simulink subsystem "microController"  (R2022b)
settings: Solver=VariableStepAuto  StartTime=0.0  StopTime=10.0  RelTol=1e-3
values from neighbouring files (symbols this model uses):
  Ts = 1/f    (= 5e-06)    [BLDCmotor.m]
  Ts_ctrl = 1/f_ctrl    (= 6.25e-05)    [BLDCmotor.m]
  vec_hallToPos = [0 2 0 1 4 3 5 0]    [BLDCmotor.m]
  Vs = motor.Vs    [BLDCmotor.m]    (also in geraModeloHover.m = 36)
libraries: slpidlib x3, spsPWMGeneratorDCDCLib x3
settings Model: Creator=hemil  LastModifiedBy=hemil

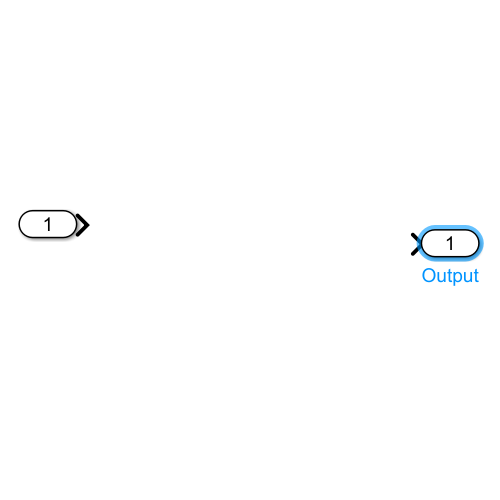
[thumbnail: Simulink's stored preview of the top-level diagram]
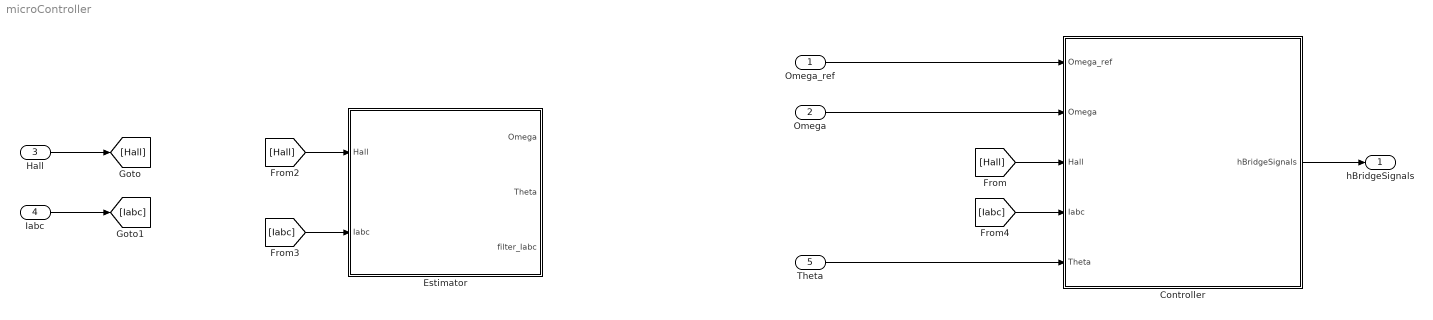
== system microController ==
  Omega_ref : Inport
  Omega : Inport  Port=2
  Hall : Inport  Port=3
  Iabc : Inport  Port=4
  Theta : Inport  Port=5
  Controller : Subsystem  Variant=on
  Estimator : Subsystem
  hBridgeSignals : Outport
  wires:
  Omega_ref/1 -> Controller/1(Omega_ref)
  Omega/1 -> Controller/2(Omega)
  Hall/1 -> [Hall]
  [Iabc] -> Controller/4(Iabc)
  Controller/1(hBridgeSignals) -> hBridgeSignals/1
  Theta/1 -> Controller/5(Theta)
  [Hall] -> Controller/3(Hall)
  [Hall] -> Estimator/1(Hall)
  Iabc/1 -> [Iabc]
  [Iabc] -> Estimator/2(Iabc)

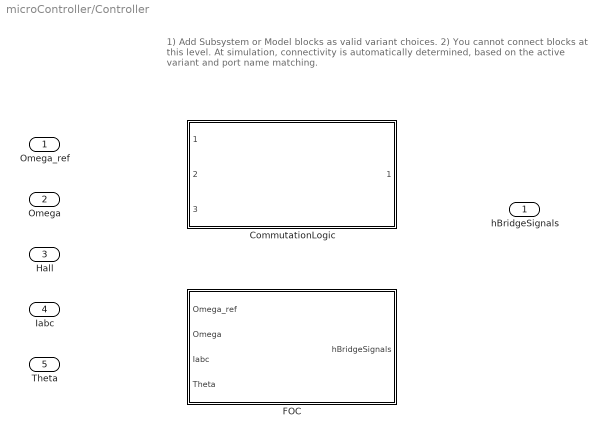
== system microController/Controller ==
  note: 1) Add Subsystem or Model blocks as valid variant choices.
      | 2) You cannot connect blocks at this level. At simulation, connectivity is automatically
      | determined, based on the active variant and port name matching.
  Omega_ref : Inport
  Omega : Inport  Port=2
  Hall : Inport  Port=3
  Iabc : Inport  Port=4
  Theta : Inport  Port=5
  CommutationLogic : Subsystem  VariantControl=(default)  ReferencedSubsystem=commutationLogic
  FOC : Subsystem  VariantControl=ControlMode == 1
  hBridgeSignals : Outport

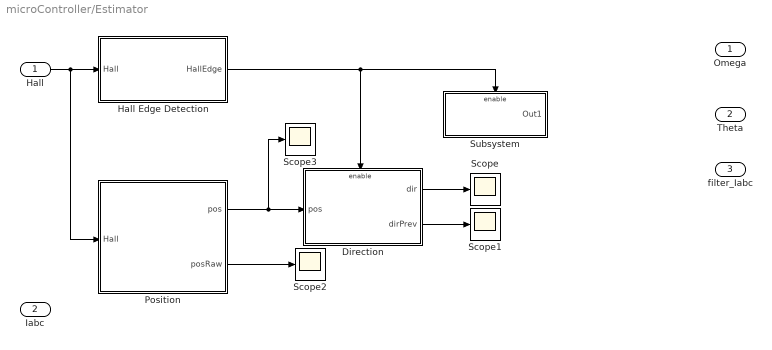
== system microController/Estimator ==
  Hall : Inport
  Iabc : Inport  Port=2
  Direction : Subsystem
  Hall Edge Detection : Subsystem
  Position : Subsystem
  Scope{,1..3} (4 alike) : Scope
  Subsystem : Subsystem
  Omega : Outport
  Theta : Outport  Port=2
  filter_Iabc : Outport  Port=3
  wires:
  Position/2(posRaw) -> Scope2/1
  Direction/2(dirPrev) -> Scope1/1
  Direction/1(dir) -> Scope/1
  Position/1(pos) -> Direction/1(pos), Scope3/1
  Hall/1 -> Hall Edge Detection/1(Hall), Position/1(Hall)
  Hall Edge Detection/1(HallEdge) -> Direction/Enable, Subsystem/Enable

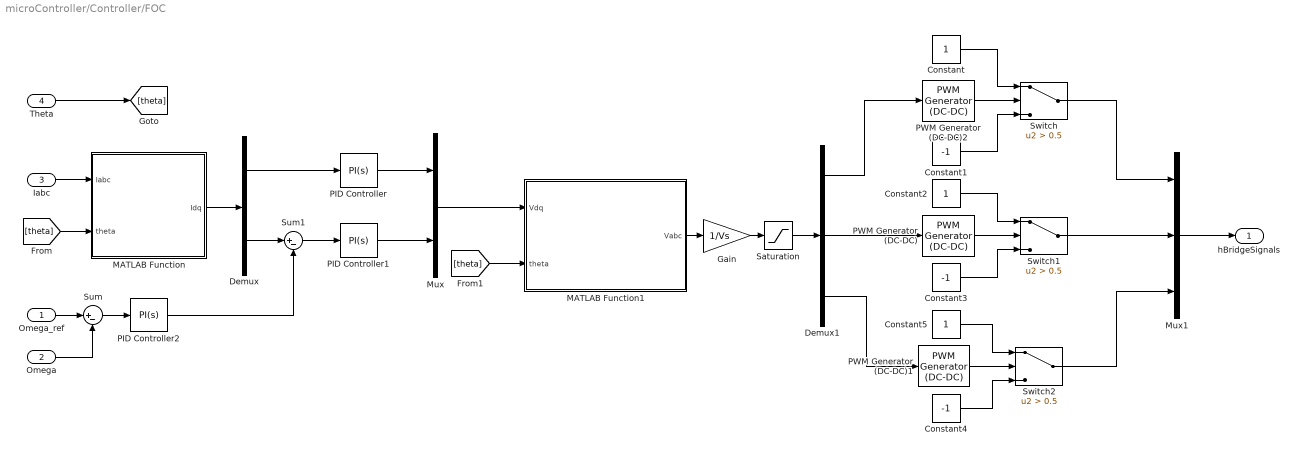
== system microController/Controller/FOC ==
  Omega_ref : Inport
  Omega : Inport  Port=2
  Iabc : Inport  Port=3
  Theta : Inport  Port=4
  Constant : Constant
  Constant1 : Constant  Value=-1
  Constant2 : Constant
  Constant3 : Constant  Value=-1
  Constant4 : Constant  Value=-1
  Constant5 : Constant
  Demux : Demux  Outputs=2
  Demux1 : Demux  Outputs=3
  Gain : Gain  Gain=1/Vs
  MATLAB Function : MATLAB Function  TreatAsAtomicUnit=on
  MATLAB Function1 : MATLAB Function  TreatAsAtomicUnit=on
  Mux : Mux  Inputs=2
  Mux1 : Mux  Inputs=3
  PID Controller : slpidlib/PID Controller  Controller=PI  Form=Parallel  TimeDomain=Continuous-time  UseExternalTs=off  SampleTime=-1  IntegratorMethod=Forward Euler  FilterMethod=Forward Euler  ControllerParametersSource=internal  P=1  I=0.1  UseKiTs=off  D=0  N=100  UseFilter=on  TunerSelectOption=Transfer Function Based (PID Tuner App)  InitialConditionSource=internal  InitialConditionForIntegrator=0  InitialConditionForFilter=0  DifferentiatorICPrevScaledInput=0  ExternalReset=none  TrackingMode=off  Kt=1  LimitOutput=off  SatLimitsSource=internal  UpperSaturationLimit=inf  LowerSaturationLimit=-inf  LinearizeAsGain=on  AntiWindupMode=none  Kb=1  LimitIntegrator=off  UpperIntegratorSaturationLimit=inf  LowerIntegratorSaturationLimit=-inf  POutMin=[]  POutMax=[]  IOutMin=[]  IOutMax=[]  DOutMin=[]  DOutMax=[]  NOutMin=[]  NOutMax=[]  SumOutMin=[]  SumOutMax=[]  SaturationOutMin=[]  SaturationOutMax=[]  PParamMin=[]  PParamMax=[]  IParamMin=[]  IParamMax=[]  DParamMin=[]  DParamMax=[]  NParamMin=[]  NParamMax=[]  KbParamMin=[]  KbParamMax=[]  KtParamMin=[]  KtParamMax=[]  KbOutMin=[]  KbOutMax=[]  KtOutMin=[]  KtOutMax=[]  IntegratorOutMin=[]  IntegratorOutMax=[]  FilterOutMin=[]  FilterOutMax=[]  SumI1OutMin=[]  SumI1OutMax=[]  SumI2OutMin=[]  SumI2OutMax=[]  SumI3OutMin=[]  SumI3OutMax=[]  SumI4OutMin=[]  SumI4OutMax=[]  SumDOutMin=[]  SumDOutMax=[]  DifferentiatorOutMin=[]  DifferentiatorOutMax=[]  FilterDiffOutCoefMin=[]  FilterDiffOutCoefMax=[]  ReciprocalOutMin=[]  ReciprocalOutMax=[]  SumDenOutMin=[]  SumDenOutMax=[]  SumNumOutMin=[]  SumNumOutMax=[]  DivideOutMin=[]  DivideOutMax=[]  UdiffTsProdOutMin=[]  UdiffTsProdOutMax=[]  NTsProdOutMin=[]  NTsProdOutMax=[]  UintegralTsProdOutMin=[]  UintegralTsProdOutMax=[]  UngainTsProdOutMin=[]  UngainTsProdOutMax=[]  ClampingZeroOutDataTypeStr=Inherit: Inherit via back propagation  ClampingZeroOutMin=[]  ClampingZeroOutMax=[]  FilterDenConstantOutDataTypeStr=Inherit: Inherit via back propagation  FilterDenConstantOutMin=[]  FilterDenConstantOutMax=[]  PCopyOutDataTypeStr=Inherit: Inherit via back propagation  PCopyOutMin=[]  PCopyOutMax=[]  NCopyOutDataTypeStr=Inherit: Inherit via back propagation  NCopyOutMin=[]  NCopyOutMax=[]  IntegratorContinuousStateAttributes=''  IntegratorStateMustResolveToSignalObject=off  IntegratorRTWStateStorageClass=Auto  FilterContinuousStateAttributes=''  FilterStateMustResolveToSignalObject=off  FilterRTWStateStorageClass=Auto  ParallelPVariant=InternalParameters  IdealPVariant=Disabled  IVariant=InternalParameters  DVariant=Disabled  IntegratorVariant=Continuous  SatVariant=Disabled  AWVariant=Passthrough  PCopyVariant=Disabled  TRVariant=Disabled  FdbkBlocksVariant=Forward  IdealPFdbkVariant=Disabled  SatFdbkVariant=Disabled  DerivativeFilterVariant=Disabled  NVariant=Disabled  NCopyVariant=Disabled_SignalSpec  FilterICVariant=Disabled  IntegratorICVariant=InternalICs  ExternalResetVariant=Disabled  TRSumVariant=Passthrough  SumFdbkVariant=Disabled  SumVariant=Sum_PI  TsampFilterVariant=InternalTs  TsampNgainVariant=Passthrough  TsampIntegralVariant=Passthrough  ExternalSaturationOutDataTypeStr=Inherit: Same as second input
  PID Controller1 : slpidlib/PID Controller  Controller=PI  Form=Parallel  TimeDomain=Continuous-time  UseExternalTs=off  SampleTime=-1  IntegratorMethod=Forward Euler  FilterMethod=Forward Euler  ControllerParametersSource=internal  P=1  I=0.1  UseKiTs=off  D=0  N=100  UseFilter=on  TunerSelectOption=Transfer Function Based (PID Tuner App)  InitialConditionSource=internal  InitialConditionForIntegrator=0  InitialConditionForFilter=0  DifferentiatorICPrevScaledInput=0  ExternalReset=none  TrackingMode=off  Kt=1  LimitOutput=off  SatLimitsSource=internal  UpperSaturationLimit=inf  LowerSaturationLimit=-inf  LinearizeAsGain=on  AntiWindupMode=none  Kb=1  LimitIntegrator=off  UpperIntegratorSaturationLimit=inf  LowerIntegratorSaturationLimit=-inf  POutMin=[]  POutMax=[]  IOutMin=[]  IOutMax=[]  DOutMin=[]  DOutMax=[]  NOutMin=[]  NOutMax=[]  SumOutMin=[]  SumOutMax=[]  SaturationOutMin=[]  SaturationOutMax=[]  PParamMin=[]  PParamMax=[]  IParamMin=[]  IParamMax=[]  DParamMin=[]  DParamMax=[]  NParamMin=[]  NParamMax=[]  KbParamMin=[]  KbParamMax=[]  KtParamMin=[]  KtParamMax=[]  KbOutMin=[]  KbOutMax=[]  KtOutMin=[]  KtOutMax=[]  IntegratorOutMin=[]  IntegratorOutMax=[]  FilterOutMin=[]  FilterOutMax=[]  SumI1OutMin=[]  SumI1OutMax=[]  SumI2OutMin=[]  SumI2OutMax=[]  SumI3OutMin=[]  SumI3OutMax=[]  SumI4OutMin=[]  SumI4OutMax=[]  SumDOutMin=[]  SumDOutMax=[]  DifferentiatorOutMin=[]  DifferentiatorOutMax=[]  FilterDiffOutCoefMin=[]  FilterDiffOutCoefMax=[]  ReciprocalOutMin=[]  ReciprocalOutMax=[]  SumDenOutMin=[]  SumDenOutMax=[]  SumNumOutMin=[]  SumNumOutMax=[]  DivideOutMin=[]  DivideOutMax=[]  UdiffTsProdOutMin=[]  UdiffTsProdOutMax=[]  NTsProdOutMin=[]  NTsProdOutMax=[]  UintegralTsProdOutMin=[]  UintegralTsProdOutMax=[]  UngainTsProdOutMin=[]  UngainTsProdOutMax=[]  ClampingZeroOutDataTypeStr=Inherit: Inherit via back propagation  ClampingZeroOutMin=[]  ClampingZeroOutMax=[]  FilterDenConstantOutDataTypeStr=Inherit: Inherit via back propagation  FilterDenConstantOutMin=[]  FilterDenConstantOutMax=[]  PCopyOutDataTypeStr=Inherit: Inherit via back propagation  PCopyOutMin=[]  PCopyOutMax=[]  NCopyOutDataTypeStr=Inherit: Inherit via back propagation  NCopyOutMin=[]  NCopyOutMax=[]  IntegratorContinuousStateAttributes=''  IntegratorStateMustResolveToSignalObject=off  IntegratorRTWStateStorageClass=Auto  FilterContinuousStateAttributes=''  FilterStateMustResolveToSignalObject=off  FilterRTWStateStorageClass=Auto  ParallelPVariant=InternalParameters  IdealPVariant=Disabled  IVariant=InternalParameters  DVariant=Disabled  IntegratorVariant=Continuous  SatVariant=Disabled  AWVariant=Passthrough  PCopyVariant=Disabled  TRVariant=Disabled  FdbkBlocksVariant=Forward  IdealPFdbkVariant=Disabled  SatFdbkVariant=Disabled  DerivativeFilterVariant=Disabled  NVariant=Disabled  NCopyVariant=Disabled_SignalSpec  FilterICVariant=Disabled  IntegratorICVariant=InternalICs  ExternalResetVariant=Disabled  TRSumVariant=Passthrough  SumFdbkVariant=Disabled  SumVariant=Sum_PI  TsampFilterVariant=InternalTs  TsampNgainVariant=Passthrough  TsampIntegralVariant=Passthrough  ExternalSaturationOutDataTypeStr=Inherit: Same as second input
  PID Controller2 : slpidlib/PID Controller  Controller=PI  Form=Parallel  TimeDomain=Continuous-time  UseExternalTs=off  SampleTime=-1  IntegratorMethod=Forward Euler  FilterMethod=Forward Euler  ControllerParametersSource=internal  P=10  I=1  UseKiTs=off  D=0  N=100  UseFilter=on  TunerSelectOption=Transfer Function Based (PID Tuner App)  InitialConditionSource=internal  InitialConditionForIntegrator=0  InitialConditionForFilter=0  DifferentiatorICPrevScaledInput=0  ExternalReset=none  TrackingMode=off  Kt=1  LimitOutput=off  SatLimitsSource=internal  UpperSaturationLimit=inf  LowerSaturationLimit=-inf  LinearizeAsGain=on  AntiWindupMode=none  Kb=1  LimitIntegrator=off  UpperIntegratorSaturationLimit=inf  LowerIntegratorSaturationLimit=-inf  POutMin=[]  POutMax=[]  IOutMin=[]  IOutMax=[]  DOutMin=[]  DOutMax=[]  NOutMin=[]  NOutMax=[]  SumOutMin=[]  SumOutMax=[]  SaturationOutMin=[]  SaturationOutMax=[]  PParamMin=[]  PParamMax=[]  IParamMin=[]  IParamMax=[]  DParamMin=[]  DParamMax=[]  NParamMin=[]  NParamMax=[]  KbParamMin=[]  KbParamMax=[]  KtParamMin=[]  KtParamMax=[]  KbOutMin=[]  KbOutMax=[]  KtOutMin=[]  KtOutMax=[]  IntegratorOutMin=[]  IntegratorOutMax=[]  FilterOutMin=[]  FilterOutMax=[]  SumI1OutMin=[]  SumI1OutMax=[]  SumI2OutMin=[]  SumI2OutMax=[]  SumI3OutMin=[]  SumI3OutMax=[]  SumI4OutMin=[]  SumI4OutMax=[]  SumDOutMin=[]  SumDOutMax=[]  DifferentiatorOutMin=[]  DifferentiatorOutMax=[]  FilterDiffOutCoefMin=[]  FilterDiffOutCoefMax=[]  ReciprocalOutMin=[]  ReciprocalOutMax=[]  SumDenOutMin=[]  SumDenOutMax=[]  SumNumOutMin=[]  SumNumOutMax=[]  DivideOutMin=[]  DivideOutMax=[]  UdiffTsProdOutMin=[]  UdiffTsProdOutMax=[]  NTsProdOutMin=[]  NTsProdOutMax=[]  UintegralTsProdOutMin=[]  UintegralTsProdOutMax=[]  UngainTsProdOutMin=[]  UngainTsProdOutMax=[]  ClampingZeroOutDataTypeStr=Inherit: Inherit via back propagation  ClampingZeroOutMin=[]  ClampingZeroOutMax=[]  FilterDenConstantOutDataTypeStr=Inherit: Inherit via back propagation  FilterDenConstantOutMin=[]  FilterDenConstantOutMax=[]  PCopyOutDataTypeStr=Inherit: Inherit via back propagation  PCopyOutMin=[]  PCopyOutMax=[]  NCopyOutDataTypeStr=Inherit: Inherit via back propagation  NCopyOutMin=[]  NCopyOutMax=[]  IntegratorContinuousStateAttributes=''  IntegratorStateMustResolveToSignalObject=off  IntegratorRTWStateStorageClass=Auto  FilterContinuousStateAttributes=''  FilterStateMustResolveToSignalObject=off  FilterRTWStateStorageClass=Auto  ParallelPVariant=InternalParameters  IdealPVariant=Disabled  IVariant=InternalParameters  DVariant=Disabled  IntegratorVariant=Continuous  SatVariant=Disabled  AWVariant=Passthrough  PCopyVariant=Disabled  TRVariant=Disabled  FdbkBlocksVariant=Forward  IdealPFdbkVariant=Disabled  SatFdbkVariant=Disabled  DerivativeFilterVariant=Disabled  NVariant=Disabled  NCopyVariant=Disabled_SignalSpec  FilterICVariant=Disabled  IntegratorICVariant=InternalICs  ExternalResetVariant=Disabled  TRSumVariant=Passthrough  SumFdbkVariant=Disabled  SumVariant=Sum_PI  TsampFilterVariant=InternalTs  TsampNgainVariant=Passthrough  TsampIntegralVariant=Passthrough  ExternalSaturationOutDataTypeStr=Inherit: Same as second input
  PWM Generator (DC-DC) : spsPWMGeneratorDCDCLib/PWM Generator (DC-DC)  Fsw=16000  Ts=0
  PWM Generator (DC-DC)1 : spsPWMGeneratorDCDCLib/PWM Generator (DC-DC)  Fsw=16000  Ts=0
  PWM Generator (DC-DC)2 : spsPWMGeneratorDCDCLib/PWM Generator (DC-DC)  Fsw=16000  Ts=0
  Saturation : Saturate  UpperLimit=1  LowerLimit=0
  Sum : Sum  Inputs=|+-
  Sum1 : Sum  Inputs=|+-
  Switch : Switch  Criteria=u2 > Threshold  Threshold=0.5  SaturateOnIntegerOverflow=off  InputSameDT=off
  Switch1 : Switch  Criteria=u2 > Threshold  Threshold=0.5  SaturateOnIntegerOverflow=off  InputSameDT=off
  Switch2 : Switch  Criteria=u2 > Threshold  Threshold=0.5  SaturateOnIntegerOverflow=off  InputSameDT=off
  hBridgeSignals : Outport
  wires:
  Gain/1 -> Saturation/1
  MATLAB Function1/1(Vabc) -> Gain/1
  Saturation/1 -> Demux1/1
  Mux1/1 -> hBridgeSignals/1
  Switch2/1 -> Mux1/3
  Switch1/1 -> Mux1/2
  Switch/1 -> Mux1/1
  Constant5/1 -> Switch2/1
  Constant4/1 -> Switch2/3
  Constant3/1 -> Switch1/3
  Constant2/1 -> Switch1/1
  Constant/1 -> Switch/1
  Constant1/1 -> Switch/3
  PWM Generator (DC-DC)1/1 -> Switch2/2
  PWM Generator (DC-DC)/1 -> Switch1/2
  PWM Generator (DC-DC)2/1 -> Switch/2
  Demux1/1 -> PWM Generator (DC-DC)2/1
  Demux1/3 -> PWM Generator (DC-DC)1/1
  Demux1/2 -> PWM Generator (DC-DC)/1
  Mux/1 -> MATLAB Function1/1(Vdq)
  PID Controller1/1 -> Mux/2
  PID Controller/1 -> Mux/1
  [theta] -> MATLAB Function1/2(theta)
  [theta] -> MATLAB Function/2(theta)
  Theta/1 -> [theta]
  Sum1/1 -> PID Controller1/1
  PID Controller2/1 -> Sum1/2
  Demux/2 -> Sum1/1
  Sum/1 -> PID Controller2/1
  Omega/1 -> Sum/2
  Omega_ref/1 -> Sum/1
  Demux/1 -> PID Controller/1
  MATLAB Function/1(Idq) -> Demux/1
  Iabc/1 -> MATLAB Function/1(Iabc)

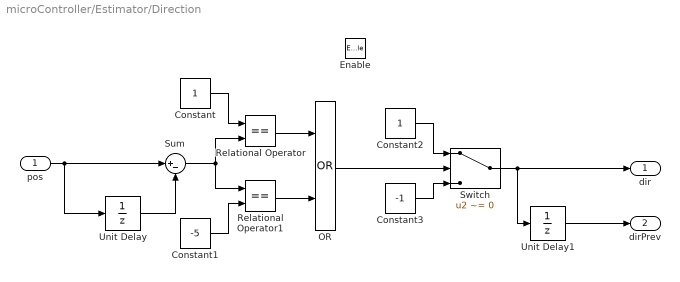
== system microController/Estimator/Direction ==
  pos : Inport
  Enable : EnablePort
  Constant : Constant
  Constant1 : Constant  Value=-5
  Constant2 : Constant
  Constant3 : Constant  Value=-1
  OR : Logic  Operator=OR  AllPortsSameDT=off  OutDataTypeStr=boolean
  Relational Operator : RelationalOperator  Operator===  OutDataTypeStr=boolean  RndMeth=Simplest  InputSameDT=off
  Relational Operator1 : RelationalOperator  Operator===  OutDataTypeStr=boolean  RndMeth=Simplest  InputSameDT=off
  Sum : Sum  Inputs=|+-
  Switch : Switch  Criteria=u2 ~= 0  SaturateOnIntegerOverflow=off  InputSameDT=off
  Unit Delay : UnitDelay  SampleTime=-1  HasFrameUpgradeWarning=on
  Unit Delay1 : UnitDelay  SampleTime=-1  HasFrameUpgradeWarning=on
  dir : Outport
  dirPrev : Outport  Port=2
  wires:
  Unit Delay1/1 -> dirPrev/1
  Constant3/1 -> Switch/3
  Constant2/1 -> Switch/1
  Switch/1 -> dir/1, Unit Delay1/1
  OR/1 -> Switch/2
  Relational Operator1/1 -> OR/2
  Relational Operator/1 -> OR/1
  Constant1/1 -> Relational Operator1/2
  Constant/1 -> Relational Operator/1
  Sum/1 -> Relational Operator/2, Relational Operator1/1
  Unit Delay/1 -> Sum/2
  pos/1 -> Unit Delay/1, Sum/1

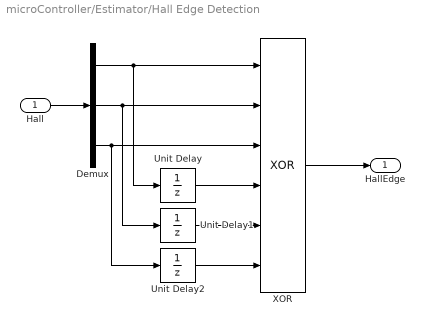
== system microController/Estimator/Hall Edge Detection ==
  Hall : Inport
  Demux : Demux  Outputs=3
  Unit Delay : UnitDelay  SampleTime=Ts_ctrl  HasFrameUpgradeWarning=on
  Unit Delay1 : UnitDelay  SampleTime=Ts_ctrl  HasFrameUpgradeWarning=on
  Unit Delay2 : UnitDelay  SampleTime=Ts_ctrl  HasFrameUpgradeWarning=on
  XOR : Logic  Operator=XOR  Inputs=6  AllPortsSameDT=off  OutDataTypeStr=boolean
  HallEdge : Outport  OutDataTypeStr=boolean
  wires:
  Unit Delay2/1 -> XOR/6
  Unit Delay1/1 -> XOR/5
  Unit Delay/1 -> XOR/4
  XOR/1 -> HallEdge/1
  Hall/1 -> Demux/1
  Demux/2 -> XOR/2, Unit Delay1/1
  Demux/3 -> XOR/3, Unit Delay2/1
  Demux/1 -> XOR/1, Unit Delay/1

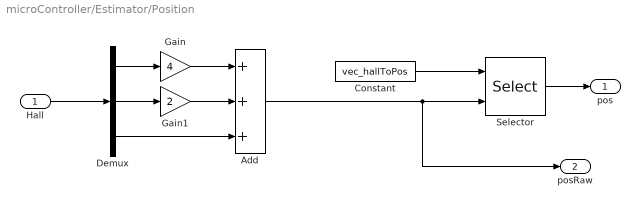
== system microController/Estimator/Position ==
  Hall : Inport
  Add : Sum  Inputs=+++
  Constant : Constant  Value=vec_hallToPos  OutDataTypeStr=int8
  Demux : Demux  Outputs=3
  Gain : Gain  Gain=4  OutDataTypeStr=uint8
  Gain1 : Gain  Gain=2  OutDataTypeStr=uint8
  Selector : Selector  IndexMode=Zero-based  InputPortWidth=length(vec_hallToPos)  IndexOptions=Index vector (port)  Indices=[1 3]  OutputSizes=1
  pos : Outport
  posRaw : Outport  Port=2
  wires:
  Hall/1 -> Demux/1
  Selector/1 -> pos/1
  Demux/1 -> Gain/1
  Constant/1 -> Selector/1
  Demux/3 -> Add/3
  Add/1 -> Selector/2, posRaw/1
  Gain/1 -> Add/1
  Gain1/1 -> Add/2
  Demux/2 -> Gain1/1

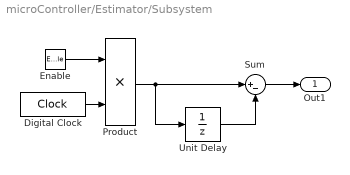
== system microController/Estimator/Subsystem ==
  Enable : EnablePort  ShowOutputPort=on
  Digital Clock : DigitalClock  SampleTime=Ts
  Product : Product
  Sum : Sum  Inputs=|+-
  Unit Delay : UnitDelay  SampleTime=Ts  HasFrameUpgradeWarning=on
  Out1 : Outport  SampleTime=Ts  InitialOutput=0
  wires:
  Sum/1 -> Out1/1
  Enable/1 -> Product/1
  Digital Clock/1 -> Product/2
  Product/1 -> Sum/1, Unit Delay/1
  Unit Delay/1 -> Sum/2

== matlab function microController/Controller/FOC/MATLAB Function1 ==
  data: Vdq input; Vabc output; theta input
function Vabc = InvClarkeParkTransform(Vdq, theta)
    %% Clarke Transform Matrix
    % Since the 3 phase currents are balanced (Ia + Ib + Ic) = 0
    % The transformation from Iabc to Ialphabeta can be reduced by
    % Ic = -Ia - Ib
    % TClarke = [   1           0;
    %           sqrt(3)/3 2*sqrt(3)/3]
    %% Augmented Park Transform
    % TPark = [ cos(theta) sin(theta);
    %          -sin(theta) cos(theta)]

    %% The matrix that realizes both the transformations are given by their product
    %TClarkePark = (2/3)*[sqrt(3)*sin(theta + pi/3), sqrt(3)*sin(theta);
    %                     sqrt(3)*cos(theta + pi/3), sqrt(3)*cos(theta)];

    %% The inverse transform is given by
    invTClarkePark = [     cos(theta),       -sin(theta);
                      -cos(theta + pi/3), sin(theta + pi/3)];

    Vab = invTClarkePark*Vdq;
    Vabc = [Vab; -sum(Vab)];

== matlab function microController/Controller/FOC/MATLAB Function ==
  data: Iabc input; Idq output; theta input
function Idq  = ClarkeParkTransform(Iabc, theta)
    %% Clarke Transform Matrix
    % Since the 3 phase currents are balanced (Ia + Ib + Ic) = 0
    % The transformation from Iabc to Ialphabeta can be reduced by
    % Ic = -Ia - Ib
    % TClarke = [   1           0;
    %           sqrt(3)/3 2*sqrt(3)/3]
    %% Augmented Park Transform
    % TPark = [ cos(theta) sin(theta);
    %          -sin(theta) cos(theta)]

    %% The matrix that realizes both the transformations are given by their product
    sqrt3 = sqrt(3);
    TClarkePark = (2/3)*[sqrt3*sin(theta + pi/3), sqrt3*sin(theta);
                         sqrt3*cos(theta + pi/3), sqrt3*cos(theta)];

    Idq = TClarkePark*Iabc(1:2);
